simulink model "et_robocon_princess_pi"  (R2013b)
settings: Solver=FixedStepDiscrete  SolverMode=SingleTasking  StartTime=0.0  StopTime=inf  FixedStep=balancer_ts  RelTol=1e-3
undefined symbols (not defined in the file): a_d, a_r, balancerStates_Bus0, Batt, battery_gain, battery_offset, cmd_max, current_mode_status, current_task_operation_status, DiscIntNeverNeededParam, exec_period, Init_Bus0, K, k_f, k_i, k_phidot, k_thetadot, lightCalib, R, see_saw_princess, STATE, TRACK_MODE_LIST, ts2, W
libraries: legonxtlib x29, simulink x19, simulink_extras x4
(part 2 of 4)

== system et_robocon_princess_pi/Main Controller/normal_operation_modes.see_saw_princess/see_saw_mode.DispVar ==
  Var : Inport  OutDataTypeStr=single  PortDimensions=1
  f : TriggerPort  TriggerType=function-call
      settings: CopyFcn=Stateflow.SLINSF.SimulinkMan.removeBlockPreDeleteFcn  PreDeleteFcn=Stateflow.SLINSF.SimulinkMan.unsafePredeleteFcn
  Gain : Gain  Gain=100
  LCD : legonxtlib/LCD  slcdStr=Light  slcdLine=5  slcdFormat=Decimal
  wires:
  Var/1 -> Gain/1
  Gain/1 -> LCD/1

== system et_robocon_princess_pi/Main Controller/normal_operation_modes.see_saw_princess/see_saw_mode.Speak ==
  f : TriggerPort  TriggerType=function-call
      settings: CopyFcn=Stateflow.SLINSF.SimulinkMan.removeBlockPreDeleteFcn  PreDeleteFcn=Stateflow.SLINSF.SimulinkMan.unsafePredeleteFcn
  Constant : Constant  Value=50
  Speaker : legonxtlib/Speaker  sinputMode=Volume only  sspeakerFreq=800  sspeakerVolume=50  sspeakerDuration=100
  wires:
  Constant/1 -> Speaker/1

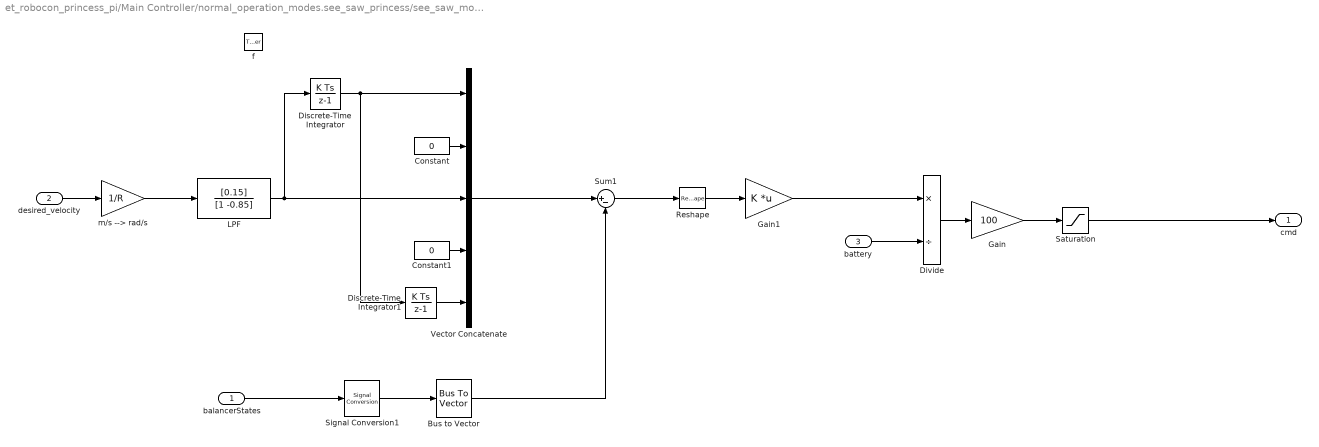
== system et_robocon_princess_pi/Main Controller/normal_operation_modes.see_saw_princess/see_saw_mode.balance_ctrl ==
  balancerStates : Inport  OutDataTypeStr=Bus: Balancer_States_Bus  PortDimensions=1
  desired_velocity : Inport  Port=2  OutDataTypeStr=single  PortDimensions=1  BusOutputAsStruct=on
  battery : Inport  Port=3  OutDataTypeStr=double  PortDimensions=1
  f : TriggerPort  TriggerType=function-call
      settings: CopyFcn=Stateflow.SLINSF.SimulinkMan.removeBlockPreDeleteFcn  PreDeleteFcn=Stateflow.SLINSF.SimulinkMan.unsafePredeleteFcn
  Bus to Vector : BusToVector
  Constant : Constant  Value=0  OutDataTypeStr=single
  Constant1 : Constant  Value=0  OutDataTypeStr=single
  Discrete-Time Integrator : DiscreteIntegrator  SampleTime=-1  ICPrevOutput=DiscIntNeverNeededParam  ICPrevScaledInput=DiscIntNeverNeededParam
  Discrete-Time Integrator1 : DiscreteIntegrator  SampleTime=-1  ICPrevOutput=DiscIntNeverNeededParam  ICPrevScaledInput=DiscIntNeverNeededParam
  Divide : Product  Inputs=*/
  Gain : Gain  Gain=100
  Gain1 : Gain  Gain=K  Multiplication=Matrix(K*u)
  LPF : DiscreteFilter  Numerator=[0.15]  Denominator=[1 -0.85]
  Reshape : Reshape  OutputDimensionality=Column vector (2-D)
  Saturation : Saturate  UpperLimit=100  LowerLimit=-100  OutDataTypeStr=single
  Signal Conversion1 : SignalConversion  ConversionOutput=Virtual bus
  Sum1 : Sum  Inputs=|+-
  Vector Concatenate : Concatenate  NumInputs=5
  m/s --> rad/s : Gain  Gain=1/R
  cmd : Outport  OutDataTypeStr=single  PortDimensions=1  InitialOutput=0
  wires:
  Reshape/1 -> Gain1/1
  Sum1/1 -> Reshape/1
  desired_velocity/1 -> m/s --> rad/s/1
  Bus to Vector/1 -> Sum1/2
  balancerStates/1 -> Signal Conversion1/1
  Vector Concatenate/1 -> Sum1/1
  battery/1 -> Divide/2
  Saturation/1 -> cmd/1
  Gain1/1 -> Divide/1
  Gain/1 -> Saturation/1
  Divide/1 -> Gain/1
  Signal Conversion1/1 -> Bus to Vector/1
  m/s --> rad/s/1 -> LPF/1
  Constant/1 -> Vector Concatenate/2
  LPF/1 -> Discrete-Time Integrator/1, Vector Concatenate/3
  Constant1/1 -> Vector Concatenate/4
  Discrete-Time Integrator/1 -> Discrete-Time Integrator1/1, Vector Concatenate/1
  Discrete-Time Integrator1/1 -> Vector Concatenate/5

== system et_robocon_princess_pi/Main Controller/normal_operation_modes.see_saw_princess/see_saw_mode.lineTracker ==
  desiredLight : Inport  OutDataTypeStr=single  PortDimensions=1
  light : Inport  Port=2  OutDataTypeStr=single  PortDimensions=1
  trackingPower : Inport  Port=3  OutDataTypeStr=single  PortDimensions=1
  battery : Inport  Port=4  OutDataTypeStr=double  PortDimensions=1
  f : TriggerPort  TriggerType=function-call
      settings: CopyFcn=Stateflow.SLINSF.SimulinkMan.removeBlockPreDeleteFcn  PreDeleteFcn=Stateflow.SLINSF.SimulinkMan.unsafePredeleteFcn
  Constant : Constant  Value=0  OutDataTypeStr=single
  Dead Zone : DeadZone  LowerValue=-0.02  UpperValue=0.02  SaturateOnIntegerOverflow=on
  Divide : Product  Inputs=*/
  Gain : Gain  Gain=100
  LPF and deriv : Subsystem
  PD : Gain  Gain="[4  0.02]/2"  Multiplication=Matrix(K*u)
  Product : Product
  Saturation : Saturate  UpperLimit=6  LowerLimit=-6
  Saturation1 : Saturate  UpperLimit=100  LowerLimit=-100  OutDataTypeStr=single
  Sum : Sum  Inputs=|+-
  Vector Concatenate : Concatenate
  Vector Concatenate1 : Concatenate
  switch side of line : Gain  Gain=-1
  cmd : Outport  OutDataTypeStr=single  PortDimensions=1
  wires:
  switch side of line/1 -> cmd/1
  desiredLight/1 -> Vector Concatenate/1
  Constant/1 -> Vector Concatenate/2  "desired light derivative"
  LPF and deriv/1(light_dot) -> Vector Concatenate1/2
  light/1 -> LPF and deriv/1(light), Vector Concatenate1/1
  Vector Concatenate/1 -> Sum/1
  Vector Concatenate1/1 -> Sum/2
  Sum/1 -> Dead Zone/1
  Dead Zone/1 -> PD/1
  PD/1 -> Saturation/1
  Saturation/1 -> Product/2
  trackingPower/1 -> Product/1
  Product/1 -> Divide/1
  battery/1 -> Divide/2
  Gain/1 -> Saturation1/1
  Divide/1 -> Gain/1
  Saturation1/1 -> switch side of line/1

== system et_robocon_princess_pi/Main Controller/normal_operation_modes.see_saw_princess/see_saw_mode.phiController ==
  phi : Inport  OutDataTypeStr=single  PortDimensions=1
  desiredPhi : Inport  Port=2  OutDataTypeStr=single  PortDimensions=1
  battery : Inport  Port=3  OutDataTypeStr=double  PortDimensions=1
  f : TriggerPort  TriggerType=function-call
      settings: CopyFcn=Stateflow.SLINSF.SimulinkMan.removeBlockPreDeleteFcn  PreDeleteFcn=Stateflow.SLINSF.SimulinkMan.unsafePredeleteFcn
  Divide : Product  Inputs=*/
  Gain : Gain  Gain=-10
  Gain1 : Gain  Gain=100
  Saturation1 : Saturate  UpperLimit=100  LowerLimit=-100  OutDataTypeStr=single
  Sum : Sum  Inputs=|+-
  cmd : Outport
  wires:
  desiredPhi/1 -> Sum/1
  phi/1 -> Sum/2
  Sum/1 -> Gain/1
  battery/1 -> Divide/2
  Gain1/1 -> Saturation1/1
  Divide/1 -> Gain1/1
  Gain/1 -> Divide/1
  Saturation1/1 -> cmd/1

== system et_robocon_princess_pi/Main Controller/normal_operation_modes.see_saw_princess/see_saw_mode.processLight ==
  rawLight : Inport  OutDataTypeStr=single  PortDimensions=1
  lightCalib : Inport  Port=2  OutDataTypeStr=Bus: Light_Bus  PortDimensions=1
  f : TriggerPort  TriggerType=function-call
      settings: CopyFcn=Stateflow.SLINSF.SimulinkMan.removeBlockPreDeleteFcn  PreDeleteFcn=Stateflow.SLINSF.SimulinkMan.unsafePredeleteFcn
  Bus Selector : BusSelector  OutputSignals=black,white
  Gain : Gain  Gain=0.3
  Gain1 : Gain  Gain=1/100
  Sum : Sum  Inputs=|+-
  Sum1 : Sum  Inputs=|++
  Sum2 : Sum  Inputs=|+-
  light : Outport
  wires:
  lightCalib/1 -> Bus Selector/1
  Bus Selector/1 -> Sum/1  "<black>"
  Bus Selector/2 -> Sum1/2, Sum/2  "<white>"
  Sum/1 -> Gain/1
  Gain/1 -> Sum1/1
  rawLight/1 -> Sum2/1
  Sum1/1 -> Sum2/2
  Sum2/1 -> Gain1/1
  Gain1/1 -> light/1

== system et_robocon_princess_pi/Main Controller/normal_operation_modes.see_saw_princess/see_saw_mode.tail_controller ==
  note: Could be improved, PI for example
  current : Inport  OutDataTypeStr=single  PortDimensions=1
  desired : Inport  Port=2  OutDataTypeStr=single  PortDimensions=1
  f : TriggerPort  TriggerType=function-call
      settings: CopyFcn=Stateflow.SLINSF.SimulinkMan.removeBlockPreDeleteFcn  PreDeleteFcn=Stateflow.SLINSF.SimulinkMan.unsafePredeleteFcn
  Gain : Gain  Gain=250
  Saturation : Saturate  UpperLimit=100  LowerLimit=-100  OutDataTypeStr=single
  Sum : Sum  Inputs=|+-
  cmd : Outport  OutDataTypeStr=single  PortDimensions=1  InitialOutput=0
  wires:
  Sum/1 -> Gain/1
  current/1 -> Sum/2
  desired/1 -> Sum/1
  Gain/1 -> Saturation/1
  Saturation/1 -> cmd/1

== system et_robocon_princess_pi/State Estimation/Data Type Conversion Unit Conversion Tail Initialization ==
  u : Inport
  init_tail : Inport  Port=2
  Bus Creator : BusCreator  Inputs=11  OutDataTypeStr=Bus: Sensors_Bus
  Bus Selector : BusSelector  OutputSignals=theta_L,theta_R,theta_T,light,gyro,sonar,battery,touch,time,ok_button,BT_status_in
  Degrees to Radians{,1..2,4} (4 alike) : simulink_extras/Transformations/Degrees to Radians
  Low Pass Filter : Subsystem
  Process Sonar : Subsystem  Commented=through
  Vmax : Subsystem
  tail processing : Subsystem
  y : Outport
  wires:
  Bus Selector/11 -> Bus Creator/11  "<BT_status_in>"
  Process Sonar/1(sonar) -> Bus Creator/6
  Bus Selector/6 -> Process Sonar/1(sonar_in)  "<sonar>"
  Bus Selector/10 -> Bus Creator/10  "<ok_button>"
  init_tail/1 -> tail processing/2(init_tail)
  Bus Selector/9 -> Bus Creator/9  "<time>"
  Bus Selector/8 -> Bus Creator/8  "<touch>"
  tail processing/1(tail) -> Bus Creator/3  "theta_T"
  Degrees to Radians4/1 -> tail processing/1(sensors)
  Vmax/1(Vmax) -> Bus Creator/7  "battery"
  Degrees to Radians2/1 -> Bus Creator/5  "gyro"
  Bus Selector/3 -> Degrees to Radians4/1  "<theta_T>"
  Bus Selector/7 -> Low Pass Filter/1(u)  "<battery>"
  Bus Selector/5 -> Degrees to Radians2/1  "<gyro>"
  Bus Selector/4 -> Bus Creator/4  "<light>"
  Bus Creator/1 -> y/1
  u/1 -> Bus Selector/1
  Degrees to Radians/1 -> Bus Creator/1  "theta_L"
  Bus Selector/2 -> Degrees to Radians1/1  "<theta_R>"
  Bus Selector/1 -> Degrees to Radians/1  "<theta_L>"
  Low Pass Filter/1(y) -> Vmax/1(Battery)  "battery"
  Degrees to Radians1/1 -> Bus Creator/2  "theta_R"

== system et_robocon_princess_pi/State Estimation/Fall Detection ==
  gyro : Inport
      settings: AttributesFormatString=Output data type: %<OutDataTypeStr>
  reset : Inport  Port=2  OutDataTypeStr=boolean
      settings: AttributesFormatString=Output data type: %<OutDataTypeStr>
  Abs : Abs
  Compare To Constant : simulink/Logic and Bit Operations/Compare To Constant  relop=>  const=1  OutDataTypeStr=boolean
  Terminator : Terminator
  aggregate_fall_detection_comparison : Logic  Operator=OR  OutDataTypeStr=boolean
  boolean_to_integer_conversion : DataTypeConversion  OutDataTypeStr=uint8
      settings: AttributesFormatString=Output data type: %<OutDataTypeStr>
  previous_fall_detection_status : UnitDelay  SampleTime=-1
  reset_output_overrice_switch : MultiPortSwitch  DataPortOrder=Zero-based contiguous  Inputs=2  zeroidx=on  InputSameDT=on
  reset_output_value : Constant  Value=false
  reset_output_value1 : Constant  Value=false  OutDataTypeStr=boolean
  fall_detected : Outport
  wires:
  reset_output_overrice_switch/1 -> Terminator/1, previous_fall_detection_status/1
  reset_output_value/1 -> reset_output_overrice_switch/3
  aggregate_fall_detection_comparison/1 -> reset_output_overrice_switch/2
  boolean_to_integer_conversion/1 -> reset_output_overrice_switch/1
  reset/1 -> boolean_to_integer_conversion/1
  previous_fall_detection_status/1 -> aggregate_fall_detection_comparison/2
  Abs/1 -> Compare To Constant/1
  gyro/1 -> Abs/1
  Compare To Constant/1 -> aggregate_fall_detection_comparison/1
  reset_output_value1/1 -> fall_detected/1

== stateflow chart et_robocon_princess_pi/Main Controller ==
  state restore
  state emergency_stop
    entry:
    debugFlag = uint16(9999);
  state normal_operation_modes
    state gyro_calibration_mode
    state light_calibration_up
    state line_tracking_mode
    state see_saw_princess
    state line_tracking_after_seesaw
    state WeShouldNotBeHere
    (default) -> (junction 12) : {
        | current_mode_status = OperationModeStatusEnum.IN_PROGRESS;
        | }
    (junction 12) -> gyro_calibration_mode [order 1] : [  current_mode == OperationModeEnum.GYRO_CALIBRATION ]
    (junction 12) -> (junction 13) [order 2]
    (junction 13) -> ? [order 1] : [ current_mode == OperationModeEnum.LIGHT_CALIBRATION_ON_TAIL ]
    (junction 13) -> (junction 144) [order 1]
    (junction 144) -> light_calibration_up [order 1] : [ current_mode == OperationModeEnum.LIGHT_CALIBRATION_UP ]
    (junction 144) -> (junction 14) [order 2]
    (junction 14) -> line_tracking_mode [order 1] : [ current_mode == OperationModeEnum.LINE_TRACKING ]
    (junction 14) -> (junction 15) [order 2]
    (junction 15) -> see_saw_princess [order 1] : [ current_mode == OperationModeEnum.SEE_SAW_PRINCESS ]
    (junction 15) -> (junction 17) [order 2]
    (junction 17) -> ? [order 1] : [  current_mode == OperationModeEnum.LIMBO ]
    (junction 17) -> (junction 19) [order 1]
    (junction 19) -> ? [order 1] : [ current_mode == OperationModeEnum.LIGHT_CALIBRATION_LIMBO ]
    (junction 19) -> (junction 140) [order 1]
    (junction 140) -> line_tracking_after_seesaw [order 1] : [ current_mode == OperationModeEnum.LINE_TRACKING_ON_MAP ]
    (junction 140) -> (junction 154) [order 2]
    (junction 154) -> ? [order 1] : [ current_mode == OperationModeEnum.YOSHI ]
    (junction 154) -> (junction 99) [order 1]
    (junction 99) -> WeShouldNotBeHere
  (default) -> (junction 38) : {initFlags = Init_Bus0;BT_status_out = single(0)}
  (junction 37) -> (junction 38)
  (junction 43) -> (junction 37)
  (junction 38) -> (junction 39) : { current_mode_index = uint8( 0 ); }
  (junction 40) -> (junction 39)
  restore -> (junction 40) : [ false == touch ]
  (junction 39) -> (junction 41) : {
      | current_mode_status = OperationModeStatusEnum.NOT_STARTED;
      | }
  normal_operation_modes -> (junction 40) [order 2] : [ current_mode_status == OperationModeStatusEnum.SUCCESSFULLY_COMPLETED ]
  (junction 42) -> (junction 41)
  (junction 41) -> (junction 44) : { current_mode_index = current_mode_index + uint8( 1 ); }
  (junction 47) -> (junction 42)
  emergency_stop -> restore : [ true == touch ]
  (junction 44) -> (junction 43) [order 1] : [ numel( TRACK_MODE_LIST ) < current_mode_index ]
      | % If the "current_mode_index" has exceeded the number
      | % of elements in the list, it should "wrap" back to the start.
  (junction 44) -> (junction 45) [order 2]
  (junction 45) -> (junction 46) : {
      | current_mode = TRACK_MODE_LIST( current_mode_index );
      | }
  (junction 46) -> (junction 47) [order 1] : [  current_mode == OperationModeEnum.SKIP ]
  (junction 46) -> normal_operation_modes [order 2]
  normal_operation_modes -> emergency_stop [order 1] : [ true == fall_detection_input ]
      | {current_mode_status = OperationModeStatusEnum.ABORTED;}
  data: rawSensors input Bus: Sensors_Bus size=1; PWM output Bus: PWM_bus size=1; TRACK_MODE_LIST parameter Enum: OperationModeEnum; current_mode_index local uint8; current_mode data_store_memory; states input Bus: States_Bus size=1; fall_detection_input input boolean size=1; current_mode_status data_store_memory; sensors input Bus: Sensors_Bus size=1; lightCalib data_store_memory; debugFlag output uint16 size=1; BT_status_out output single size=1; touch input single size=1; initFlags output Bus: Init_Bus size=1; Init_Bus0 parameter Bus: Init_Bus size=1; balancerStates_Bus0 parameter Bus: Balancer_States_Bus size=1

== stateflow chart et_robocon_princess_pi/Main Controller/normal_operation_modes.light_calibration_up ==
  state wait
    entry:debugFlag = uint16(200);
  state MoveUp
    entry:debugFlag = uint16(201);
    PWM.tail = single(-50);
  state Reset
    entry:debugFlag = uint16(202);
    PWM.tail = single(0);
    initFlags.tail = single(1);
    exit:
    initFlags.tail = single(0);
    desired_tail = single(0);
  state light_sensor_calibration_up
    %during, exit: PWM.tail = tail_controller(sensors.theta_T,single(1.6))
    state WaitForBlack
      entry: debugFlag = uint16(310);
    state StoreBlack
      entry: lightCalib.black = sensors.light;
      debugFlag = uint16(311);
    state WaitForWhite
      entry: debugFlag = uint16(312)
    state StoreWhite
      entry: lightCalib.white = sensors.light;
      debugFlag = uint16(313);
    state CalibComplete
      entry:
      debugFlag = uint16(318);
      current_task_operation_status = OperationModeStatusEnum.SUCCESSFULLY_COMPLETED;
    state cmd = tail_controller(current,desired) [function]
    (default) -> WaitForBlack
    WaitForBlack -> StoreBlack : [hasChangedFrom(touch,single(0))]
    StoreBlack -> WaitForWhite : after(1,sec)
    WaitForWhite -> StoreWhite : [hasChangedFrom(touch,single(0))]
    StoreWhite -> CalibComplete : after(1,sec)
  (default) -> wait
  wait -> MoveUp : [hasChangedFrom(touch,single(0))]
  MoveUp -> Reset : after(2,sec)
  Reset -> light_sensor_calibration_up : after(1,sec)
  data: current function_input single size=1; desired function_input single size=1; cmd function_output single size=1; sensors input Bus: Sensors_Bus size=1; lightCalib data_store_memory; current_task_operation_status data_store_memory; debugFlag output uint16; touch input single size=1; PWM output Bus: PWM_bus size=1; initFlags output Bus: Init_Bus size=1; desired_tail local

== stateflow chart et_robocon_princess_pi/Main Controller/normal_operation_modes.gyro_calibration_mode ==
  state gyro_calibration_mode
    state GyroCalibration
      entry:
      desired_tail = single(1.6);
      during, exit:
      PWM.tail = tail_controller(sensors.theta_T,desired_tail);
      state MoveTailDown
        entry:
        debugFlag = uint16(204);
        during:
        desired_tail = desired_tail + single(0.008);
      state StartCalibration
        entry:
        debugFlag = uint16(205);
        initFlags.gyroInit = single(1);
        initFlags.gyroReset = single(1);
        initFlags.theta = single(1);
      state Wait
        entry: Speak;
      state MakeNoise
        during: Speak;
      state StartCalibration1
        entry:
        debugFlag = uint16(208);
        initFlags.gyroInit = single(0);
        initFlags.gyroReset = single(0);
        initFlags.theta = single(0);
      state CalibComplete
        entry:
        debugFlag = uint16(209);
        current_task_operation_status = OperationModeStatusEnum.SUCCESSFULLY_COMPLETED;
      state cmd = tail_controller(current,desired) [function]
      state Speak [function]
      (default) -> StartCalibration
      MoveTailDown -> StartCalibration : [desired_tail >= single(1.6) ]
      StartCalibration -> Wait : [hasChangedFrom(touch,single(0))]
      Wait -> MakeNoise : after(5,sec)
      MakeNoise -> StartCalibration1 : after(0.5,sec)
      StartCalibration1 -> CalibComplete
    (default) -> GyroCalibration
  data: current function_input single size=1; desired function_input single size=1; cmd function_output single size=1; debugFlag output uint16 size=1; current_task_operation_status data_store_memory; sensors input Bus: Sensors_Bus size=1; touch input single size=1; initFlags output Bus: Init_Bus size=1; PWM output Bus: PWM_bus size=1; desired_tail local

== system et_robocon_princess_pi/State Estimation/Gyro Processing ==
  sensors : Inport
  gyroInit : Inport  Port=2
  gyroReset : Inport  Port=3
  Bus Selector1 : BusSelector  OutputSignals=gyro
  Compute psi : Subsystem
  Gyro initialization : Subsystem  TreatAsAtomicUnit=on
  Reset Subsystem : Stateflow chart  TreatAsAtomicUnit=on
  Sum : Sum  Inputs=-+|
  psi : Outport
  psi_dot : Outport  Port=2
  psi filtered : Outport  Port=3
  wires:
  Compute psi/2(Filtered) -> psi filtered/1
  Reset Subsystem/1(doProcess()) -> Compute psi/Trigger
  gyroReset/1 -> Reset Subsystem/1(init_flag)
  Bus Selector1/1 -> Sum/2, Gyro initialization/1(gyro)  "<gyro>"
  Gyro initialization/1(psi_dot_0) -> Sum/1
  Sum/1 -> psi_dot/1, Compute psi/1(gyro)
  Compute psi/1(psi) -> psi/1
  sensors/1 -> Bus Selector1/1
  gyroInit/1 -> Gyro initialization/Enable

== system et_robocon_princess_pi/State Estimation/StateEstimation ==
  note: Conversion from Raw Sensors to States as described in "NXTway plant model.pdf"
  Sensors : Inport
  psi : Inport  Port=2
  psi_dot : Inport  Port=3
  init theta : Inport  Port=4
  Bus Creator1 : BusCreator  OutDataTypeStr=Bus: States_Bus
  Bus Creator2 : BusCreator  Inputs=5  OutDataTypeStr=Bus: Balancer_States_Bus
  Bus Selector1 : BusSelector  OutputSignals=theta_L,theta_R
  Process theta1 : Subsystem
  Reset Subsystem : Stateflow chart  TreatAsAtomicUnit=on
  states : Outport  OutputWhenDisabled=reset  InitialOutput=0
  wires:
  Process theta1/2(psi_out) -> Bus Creator2/2  "psi"
  Reset Subsystem/1(doProcess()) -> Process theta1/Trigger
  Bus Selector1/2 -> Process theta1/3(theta_r)  "<theta_R>"
  Bus Selector1/1 -> Process theta1/2(theta_l)  "<theta_L>"
  init theta/1 -> Reset Subsystem/1(init_flag)
  Process theta1/1(theta) -> Bus Creator2/1
  Process theta1/3(theta_dot) -> Bus Creator2/3
  Process theta1/4(int_theta) -> Bus Creator2/5
  psi_dot/1 -> Bus Creator2/4  "psi_dot"
  Process theta1/6(phi_dot) -> Bus Creator1/3  "phi_dot"
  Bus Creator2/1 -> Bus Creator1/1  "balancerStates"
  Process theta1/5(phi) -> Bus Creator1/2  "phi"
  Sensors/1 -> Bus Selector1/1
  psi/1 -> Process theta1/1(psi)
  Bus Creator1/1 -> states/1
  Process theta1/7(theta_dot_dot) -> Bus Creator1/4  "theta_dot_dot"

== system et_robocon_princess_pi/Hardware/Receive Bluetooth Status/BluetoothOFF ==
  Constant : Constant  Value=single(0)
  BT_status_in : Outport
  wires:
  Constant/1 -> BT_status_in/1

== system et_robocon_princess_pi/Hardware/Receive Bluetooth Status/BluetoothONMario ==
  Data Type Conversion9 : DataTypeConversion  OutDataTypeStr=single
  Rate Transition2 : RateTransition  OutPortSampleTime=0.004
  Receive via Bluetooth(R) Connection : legonxtlib/Receive via Bluetooth(R) Connection  mailbox=3  dataType=uint8  dataSize=1  sampleTime=0.1
  Terminator : Terminator
  BT_status_in : Outport
  wires:
  Data Type Conversion9/1 -> BT_status_in/1
  Rate Transition2/1 -> Data Type Conversion9/1
  Receive via Bluetooth(R) Connection/1 -> Rate Transition2/1
  Receive via Bluetooth(R) Connection/2 -> Terminator/1

== system et_robocon_princess_pi/Hardware/Receive Bluetooth Status/BluetoothONPrincess ==
  Data Type Conversion9 : DataTypeConversion  OutDataTypeStr=single
  Rate Transition2 : RateTransition  OutPortSampleTime=0.004
  Receive via Bluetooth(R) Connection : legonxtlib/Receive via Bluetooth(R) Connection  mailbox=3  dataType=uint8  dataSize=1  sampleTime=0.1
  Terminator : Terminator
  BT_status_in : Outport
  wires:
  Receive via Bluetooth(R) Connection/2 -> Terminator/1
  Receive via Bluetooth(R) Connection/1 -> Rate Transition2/1
  Rate Transition2/1 -> Data Type Conversion9/1
  Data Type Conversion9/1 -> BT_status_in/1

== system et_robocon_princess_pi/Hardware/Send Bluetooth Status/BluetoothOFF ==
  BT_status_out : Inport
  Terminator : Terminator
  wires:
  BT_status_out/1 -> Terminator/1

== system et_robocon_princess_pi/Hardware/Send Bluetooth Status/BluetoothONMario ==
  BT_status_out : Inport
  Data Type Conversion1 : DataTypeConversion  OutDataTypeStr=uint8
  Rate Transition1 : RateTransition  OutPortSampleTime=0.1
  Send via Bluetooth(R) Connection : legonxtlib/Send via Bluetooth(R) Connection  mailbox=2
  wires:
  BT_status_out/1 -> Rate Transition1/1
  Rate Transition1/1 -> Data Type Conversion1/1
  Data Type Conversion1/1 -> Send via Bluetooth(R) Connection/1

== system et_robocon_princess_pi/Hardware/Send Bluetooth Status/BluetoothONPrincess ==
  BT_status_out : Inport
  Data Type Conversion1 : DataTypeConversion  OutDataTypeStr=uint8
  Rate Transition1 : RateTransition  OutPortSampleTime=0.1
  Send via Bluetooth(R) Connection : legonxtlib/Send via Bluetooth(R) Connection  mailbox=4
  wires:
  Data Type Conversion1/1 -> Send via Bluetooth(R) Connection/1
  Rate Transition1/1 -> Data Type Conversion1/1
  BT_status_out/1 -> Rate Transition1/1

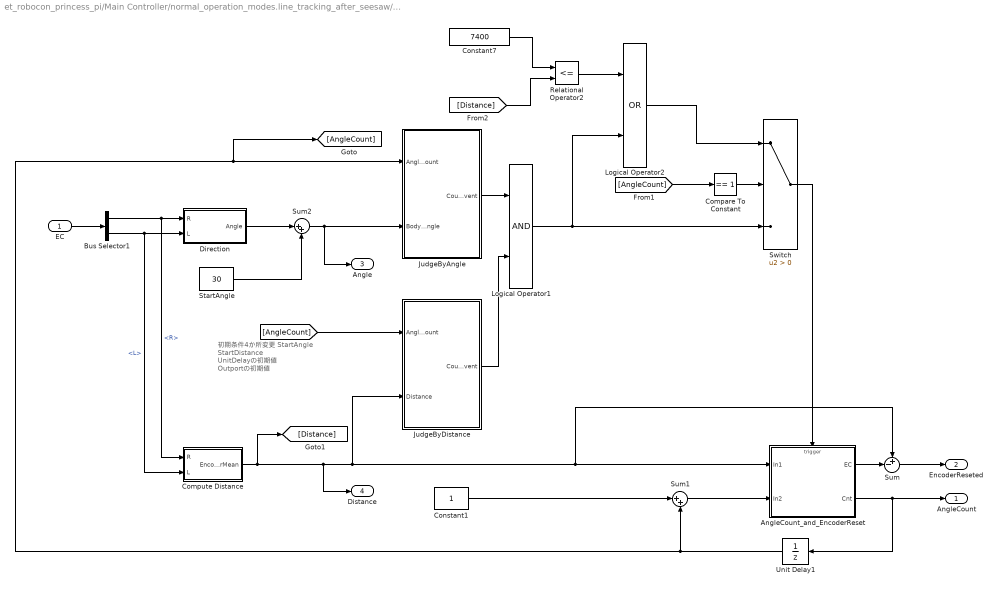
== system et_robocon_princess_pi/Main Controller/normal_operation_modes.line_tracking_after_seesaw/line_tracking_mode.Track.analyzeEncoders/AngleCounter ==
  note: 初期条件4か所変更
      | StartAngle
      | StartDistance
      | UnitDelayの初期値
      | Outportの初期値
  EC : Inport
  AngleCount_and_EncoderReset : Subsystem  TreatAsAtomicUnit=on
  Bus Selector1 : BusSelector  OutputSignals=R,L
  Compare To Constant : simulink/Logic and Bit Operations/Compare To Constant  relop===  const=1  OutDataTypeStr=boolean
  Compute Distance : Subsystem
  Constant1 : Constant  OutDataTypeStr=uint8
  Constant7 : Constant  Value=7400  OutDataTypeStr=int32
  Direction : Subsystem
  JudgeByAngle : Subsystem
  JudgeByDistance : Subsystem
  Logical Operator1 : Logic  AllPortsSameDT=off  OutDataTypeStr=boolean
  Logical Operator2 : Logic  Operator=OR  AllPortsSameDT=off  OutDataTypeStr=boolean
  Relational Operator2 : RelationalOperator  Operator=<=  OutDataTypeStr=boolean
  StartAngle : Constant  Value=30  OutDataTypeStr=int16
  Sum : Sum  Inputs=+-|
  Sum1 : Sum  Inputs=|++  AccumDataTypeStr=uint8
  Sum2 : Sum  Inputs=|++
  Switch : Switch  Criteria=u2 > Threshold
  Unit Delay1 : UnitDelay  InitialCondition=1  SampleTime=-1
  AngleCount : Outport
  EncoderReseted : Outport  Port=2
  Angle : Outport  Port=3
  Distance : Outport  Port=4
  wires:
  Sum2/1 -> JudgeByAngle/2(BodyAngle), Angle/1
  Sum1/1 -> AngleCount_and_EncoderReset/2(In2)
  Constant1/1 -> Sum1/1
  Unit Delay1/1 -> [AngleCount], JudgeByAngle/1(AngleCount), Sum1/2
  AngleCount_and_EncoderReset/2(Cnt) -> AngleCount/1, Unit Delay1/1
  Bus Selector1/1 -> Compute Distance/1(R), Direction/1(R)  "<R>"
  Bus Selector1/2 -> Compute Distance/2(L), Direction/2(L)  "<L>"
  EC/1 -> Bus Selector1/1
  AngleCount_and_EncoderReset/1(EC) -> Sum/2
  Sum/1 -> EncoderReseted/1
  Compute Distance/1(EncoderMean) -> [Distance], Distance/1, JudgeByDistance/2(Distance), Sum/1, AngleCount_and_EncoderReset/1(In1)
  [AngleCount] -> JudgeByDistance/1(AngleCount)
  JudgeByAngle/1(CountEvent) -> Logical Operator1/1
  JudgeByDistance/1(CountEvent) -> Logical Operator1/2
  Direction/1(Angle) -> Sum2/1
  StartAngle/1 -> Sum2/2
  Logical Operator1/1 -> Logical Operator2/2, Switch/3
  Switch/1 -> AngleCount_and_EncoderReset/Trigger
  Compare To Constant/1 -> Switch/2
  [AngleCount] -> Compare To Constant/1
  Logical Operator2/1 -> Switch/1
  Constant7/1 -> Relational Operator2/1
  Relational Operator2/1 -> Logical Operator2/1
  [Distance] -> Relational Operator2/2

== system et_robocon_princess_pi/Main Controller/normal_operation_modes.line_tracking_after_seesaw/line_tracking_mode.Track.analyzeEncoders/Store x0 ==
  In1 : Inport
  In2 : Inport  Port=2
  Enable : EnablePort
  Out1 : Outport
  Out2 : Outport  Port=2
  wires:
  In1/1 -> Out1/1
  In2/1 -> Out2/1

== system et_robocon_princess_pi/Main Controller/normal_operation_modes.line_tracking_after_seesaw/line_tracking_mode.Track.lineTracker/Handler ==
  steering : Inport
  fwd : Inport  Port=2
  Constant1 : Constant  Value=-1  OutDataTypeStr=int8
  Mux : Mux  Inputs=2
  Switch1 : Switch  OutDataTypeStr=single  RndMeth=Simplest
  rocket_start : Subsystem
  slow_start : Subsystem
  cmd : Outport
  wires:
  steering/1 -> Mux/2  "str"
  slow_start/1(fwd_slow) -> Switch1/1
  Mux/1 -> cmd/1
  fwd/1 -> rocket_start/1(fwd), slow_start/1(fwd)  "fwd"
  Constant1/1 -> Switch1/2
  rocket_start/1(fwd_slow) -> Switch1/3
  Switch1/1 -> Mux/1

== system et_robocon_princess_pi/Main Controller/normal_operation_modes.line_tracking_after_seesaw/line_tracking_mode.Track.lineTracker/SwitchForFreeSteering ==
  note: Edge Change
      | -1: Run right edge
      | 1: Run left edge
  note: Target Value
  FlagSteering : Inport
  PID : Inport  Port=2  PortDimensions=5
  LightSens : Inport  Port=3
  Add : Sum  Inputs=+-  AccumDataTypeStr=single  OutDataTypeStr=single  RndMeth=Simplest
  AdjustForUnit : Gain  Gain=18.25  OutDataTypeStr=single  RndMeth=Simplest
  Constant2 : Constant  OutDataTypeStr=single  SampleTime=-1
  Constant6 : Constant  Value=0.5  OutDataTypeStr=single  SampleTime=-1
  DeleteDummyData : Selector  InputPortWidth=5  IndexOptions=Index vector (dialog)  Indices=1  OutputSizes=1
  Product1 : Product  OutDataTypeStr=single  RndMeth=Simplest
  Switch : Switch  Criteria=u2 > Threshold
  tmpController : Subsystem  TreatAsAtomicUnit=on  mask(tmp PID Controller){Ts_=ts2, SaturationMax=100, SaturationMin=-100}
      mask prompts: Ts_ "Sampling Time (Task Period)"; SaturationMax "Saturation Max Value of PID Ctrl"; SaturationMin "Saturation Min Value of PID"
      mask help:
      | Sampling Time: Task Period
      | P: Proportional Gain
      | I: Integral Gain
      | D: Derivative Gain
      | B: Back Gain for Integrator
      | Saturation Max Value of PID ctrl:
      |    Saturation Max Value of PID ctrl > Saturation Min Value of PID ctrl
      | Saturation Min Value of PID ctrl:
      |    Saturation Min Value of PID ctrl < Saturation Max Value of PID ctrl
      settings: RTWSystemCode=Inline
      mask Display: disp('PID')
  Steering : Outport
  wires:
  PID/1 -> tmpController/2(BD), DeleteDummyData/1
  Switch/1 -> Steering/1
  DeleteDummyData/1 -> Switch/1  "FreeSteering"
  FlagSteering/1 -> Switch/2
  Add/1 -> Product1/1
  LightSens/1 -> Add/1
  Constant6/1 -> Add/2
  Constant2/1 -> Product1/2
  Product1/1 -> tmpController/1(Error)  "Diff_Between_Target_and_Value"
  tmpController/1(Target_deg) -> AdjustForUnit/1
  AdjustForUnit/1 -> Switch/3  "LintTraceSteering"

== system et_robocon_princess_pi/Main Controller/normal_operation_modes.line_tracking_after_seesaw/line_tracking_mode.Track.processLight/OFF2ON ==
  In1 : Inport
  Trigger : TriggerPort
  Light Sensor Switch ON : S-Function  FunctionName=sfun_light_sw  Parameters=-1,ip,sw  EnableBusSupport=off  mask(Light Sensor ON/OFF Switch){ip=S3, sw=ON}
      mask prompts: ip "port:"; sw "switch"
      mask help: LEGO Mindstorms NXT Light Sensor switch.
      mask init:
      | [data, map]=imread('LIGHT_SENSOR.gif');
      | pic=ind2rgb(data,map);
      mask TypeOptions ip: S1 | S2 | S3 | S4
      mask TypeOptions sw: ON | OFF
      mask Display:
      | image(pic)
      | color('red')
      | fprintf('%s, %s',ip,sw)
  Out1 : Outport
  wires:
  In1/1 -> Out1/1

== system et_robocon_princess_pi/Main Controller/normal_operation_modes.line_tracking_after_seesaw/line_tracking_mode.Track.processLight/ON2OFF ==
  In1 : Inport
  Trigger : TriggerPort  TriggerType=falling
  Light Sensor Switch OFF : S-Function  FunctionName=sfun_light_sw  Parameters=-1,ip,sw  EnableBusSupport=off  mask(Light Sensor ON/OFF Switch){ip=S3, sw=OFF}
      mask prompts: ip "port:"; sw "switch"
      mask help: LEGO Mindstorms NXT Light Sensor switch.
      mask init:
      | [data, map]=imread('LIGHT_SENSOR.gif');
      | pic=ind2rgb(data,map);
      mask TypeOptions ip: S1 | S2 | S3 | S4
      mask TypeOptions sw: ON | OFF
      mask Display:
      | image(pic)
      | color('red')
      | fprintf('%s, %s',ip,sw)
  Out1 : Outport
  wires:
  In1/1 -> Out1/1

== system et_robocon_princess_pi/Main Controller/normal_operation_modes.line_tracking_after_seesaw/line_tracking_mode.balanceControl/ForSimulation ==
  cmd_forward : Inport
  cmd_turn : Inport  Port=2
  gyro : Inport  Port=3
  gyro_offset : Inport  Port=4
  theta_m_l : Inport  Port=5
  theta_m_r : Inport  Port=6
  battery : Inport  Port=7
  Cal_PWM : Subsystem
      settings: RTWSystemCode=Nonreusable function
  Cal_Reference : Subsystem  Description=|
      | 1111111111111111111
      | 2222222222222222222
      | 3333333333333333333
      | 4444444444444444444
      settings: RTWSystemCode=Nonreusable function
  Cal_x1 : Subsystem
      settings: RTWSystemCode=Nonreusable function
  DiscreteIntegrator : Subsystem
  FeedbackGain : Gain  Gain=k_f  Multiplication=Matrix(K*u)  OutDataTypeStr=Inherit: Same as input  ParamDataTypeStr=Inherit: Same as input
  IntegralGain : Gain  Gain=k_i  Multiplication=Matrix(K*u)  OutDataTypeStr=Inherit: Same as input  ParamDataTypeStr=Inherit: Same as input
  Sum1 : Sum  Inputs=|+-  OutDataTypeStr=Inherit: Same as first input
  Sum2 : Sum  Inputs=+-|  OutDataTypeStr=Inherit: Same as first input
  sum_err : Sum  Inputs=|++  OutDataTypeStr=Inherit: Same as first input
  pwm_l : Outport
  pwm_r : Outport  Port=2
  wires:
  Cal_Reference/1(pwm_turn) -> Cal_PWM/1(pwm_turn)
  cmd_turn/1 -> Cal_Reference/2(cmd_turn)
  sum_err/1 -> Cal_PWM/2(err)
  FeedbackGain/1 -> sum_err/2  "errx1"
  Cal_Reference/2(theta_ref) -> Sum1/1
  Cal_x1/1(theta) -> Sum1/2
  Sum1/1 -> DiscreteIntegrator/1(in)
  DiscreteIntegrator/1(out) -> IntegralGain/1
  IntegralGain/1 -> sum_err/1  "errtheta"
  Cal_x1/2(x1) -> Sum2/2
  Sum2/1 -> FeedbackGain/1
  Cal_Reference/3(x1_ref) -> Sum2/1
  theta_m_l/1 -> Cal_x1/3(theta_m_l)
  theta_m_r/1 -> Cal_x1/4(theta_m_r)
  cmd_forward/1 -> Cal_Reference/1(cmd_forward)
  Cal_PWM/1(pwm_l) -> pwm_l/1
  gyro/1 -> Cal_x1/1(gyro)
  Cal_PWM/2(pwm_r) -> pwm_r/1
  gyro_offset/1 -> Cal_x1/2(gyro_offset)
  battery/1 -> Cal_PWM/3(battery)

== system et_robocon_princess_pi/Main Controller/normal_operation_modes.line_tracking_after_seesaw/line_tracking_mode.balanceControl/Low Pass Filter ==
  u : Inport
  Constant : Constant  Value=0  OutDataTypeStr=boolean
  Low Pass Filter : DiscreteFilter  Numerator=[.01]  Denominator=[1 -0.99]
  Memory : Memory  X0=1  InheritSampleTime=on
  Store Offset : Subsystem  TreatAsAtomicUnit=on
  Sum1 : Sum  Inputs=++|
  Sum2 : Sum  Inputs=-+|
  y : Outport
  wires:
  Store Offset/1(x0) -> Sum1/1, Sum2/1
  u/1 -> Store Offset/1(x), Sum2/2
  Constant/1 -> Memory/1
  Memory/1 -> Store Offset/Enable
  Sum2/1 -> Low Pass Filter/1
  Sum1/1 -> y/1
  Low Pass Filter/1 -> Sum1/2

== system et_robocon_princess_pi/Main Controller/normal_operation_modes.line_tracking_after_seesaw/line_tracking_mode.balanceControl/removeOffset ==
  In1 : Inport
  In2 : Inport  Port=2
  Constant : Constant  Value=0
  Memory : Memory  X0=1  InheritSampleTime=on
  Store x0 : Subsystem  TreatAsAtomicUnit=on
  Sum : Sum  Inputs=-+|
  Sum1 : Sum  Inputs=-+|
  Out1 : Outport
  Out2 : Outport  Port=2
  wires:
  Store x0/2(Out2) -> Sum1/1
  In2/1 -> Store x0/2(In2), Sum1/2
  Constant/1 -> Memory/1
  Sum1/1 -> Out2/1
  In1/1 -> Sum/2, Store x0/1(In1)
  Store x0/1(Out1) -> Sum/1
  Memory/1 -> Store x0/Enable
  Sum/1 -> Out1/1

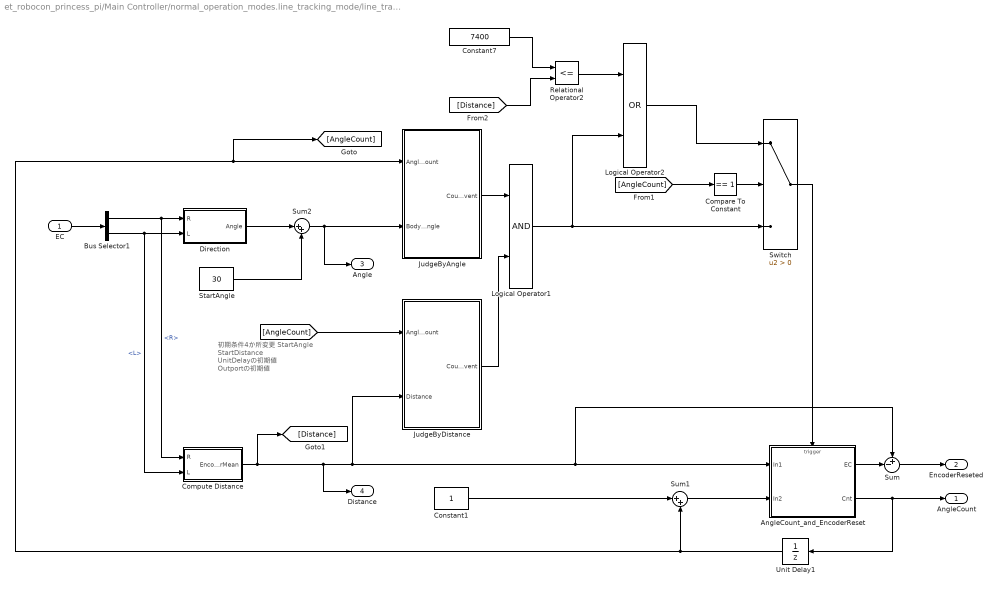
== system et_robocon_princess_pi/Main Controller/normal_operation_modes.line_tracking_mode/line_tracking_mode.Track.analyzeEncoders/AngleCounter ==
  note: 初期条件4か所変更
      | StartAngle
      | StartDistance
      | UnitDelayの初期値
      | Outportの初期値
  EC : Inport
  AngleCount_and_EncoderReset : Subsystem  TreatAsAtomicUnit=on
  Bus Selector1 : BusSelector  OutputSignals=R,L
  Compare To Constant : simulink/Logic and Bit Operations/Compare To Constant  relop===  const=1  OutDataTypeStr=boolean
  Compute Distance : Subsystem
  Constant1 : Constant  OutDataTypeStr=uint8
  Constant7 : Constant  Value=7400  OutDataTypeStr=int32
  Direction : Subsystem
  JudgeByAngle : Subsystem
  JudgeByDistance : Subsystem
  Logical Operator1 : Logic  AllPortsSameDT=off  OutDataTypeStr=boolean
  Logical Operator2 : Logic  Operator=OR  AllPortsSameDT=off  OutDataTypeStr=boolean
  Relational Operator2 : RelationalOperator  Operator=<=  OutDataTypeStr=boolean
  StartAngle : Constant  Value=30  OutDataTypeStr=int16
  Sum : Sum  Inputs=+-|
  Sum1 : Sum  Inputs=|++  AccumDataTypeStr=uint8
  Sum2 : Sum  Inputs=|++
  Switch : Switch  Criteria=u2 > Threshold
  Unit Delay1 : UnitDelay  InitialCondition=1  SampleTime=-1
  AngleCount : Outport
  EncoderReseted : Outport  Port=2
  Angle : Outport  Port=3
  Distance : Outport  Port=4
  wires:
  Sum2/1 -> JudgeByAngle/2(BodyAngle), Angle/1
  Sum1/1 -> AngleCount_and_EncoderReset/2(In2)
  Constant1/1 -> Sum1/1
  Unit Delay1/1 -> [AngleCount], JudgeByAngle/1(AngleCount), Sum1/2
  AngleCount_and_EncoderReset/2(Cnt) -> AngleCount/1, Unit Delay1/1
  Bus Selector1/1 -> Compute Distance/1(R), Direction/1(R)  "<R>"
  Bus Selector1/2 -> Compute Distance/2(L), Direction/2(L)  "<L>"
  EC/1 -> Bus Selector1/1
  AngleCount_and_EncoderReset/1(EC) -> Sum/2
  Sum/1 -> EncoderReseted/1
  Compute Distance/1(EncoderMean) -> [Distance], Distance/1, JudgeByDistance/2(Distance), Sum/1, AngleCount_and_EncoderReset/1(In1)
  [AngleCount] -> JudgeByDistance/1(AngleCount)
  JudgeByAngle/1(CountEvent) -> Logical Operator1/1
  JudgeByDistance/1(CountEvent) -> Logical Operator1/2
  Direction/1(Angle) -> Sum2/1
  StartAngle/1 -> Sum2/2
  Logical Operator1/1 -> Logical Operator2/2, Switch/3
  Switch/1 -> AngleCount_and_EncoderReset/Trigger
  Compare To Constant/1 -> Switch/2
  [AngleCount] -> Compare To Constant/1
  Logical Operator2/1 -> Switch/1
  Constant7/1 -> Relational Operator2/1
  Relational Operator2/1 -> Logical Operator2/1
  [Distance] -> Relational Operator2/2

== system et_robocon_princess_pi/Main Controller/normal_operation_modes.line_tracking_mode/line_tracking_mode.Track.lineTracker/Handler ==
  steering : Inport
  fwd : Inport  Port=2
  Constant1 : Constant  Value=-1  OutDataTypeStr=int8
  Mux : Mux  Inputs=2
  Switch1 : Switch  OutDataTypeStr=single  RndMeth=Simplest
  rocket_start : Subsystem
  slow_start : Subsystem
  cmd : Outport
  wires:
  steering/1 -> Mux/2  "str"
  slow_start/1(fwd_slow) -> Switch1/1
  Mux/1 -> cmd/1
  fwd/1 -> rocket_start/1(fwd), slow_start/1(fwd)  "fwd"
  Constant1/1 -> Switch1/2
  rocket_start/1(fwd_slow) -> Switch1/3
  Switch1/1 -> Mux/1

== system et_robocon_princess_pi/Main Controller/normal_operation_modes.line_tracking_mode/line_tracking_mode.Track.lineTracker/SwitchForFreeSteering ==
  note: Edge Change
      | -1: Run right edge
      | 1: Run left edge
  note: Target Value
  FlagSteering : Inport
  PID : Inport  Port=2  PortDimensions=5
  LightSens : Inport  Port=3
  Add : Sum  Inputs=+-  AccumDataTypeStr=single  OutDataTypeStr=single  RndMeth=Simplest
  AdjustForUnit : Gain  Gain=18.25  OutDataTypeStr=single  RndMeth=Simplest
  Constant2 : Constant  OutDataTypeStr=single  SampleTime=-1
  Constant6 : Constant  Value=0.5  OutDataTypeStr=single  SampleTime=-1
  DeleteDummyData : Selector  InputPortWidth=5  IndexOptions=Index vector (dialog)  Indices=1  OutputSizes=1
  Product1 : Product  OutDataTypeStr=single  RndMeth=Simplest
  Switch : Switch  Criteria=u2 > Threshold
  tmpController : Subsystem  TreatAsAtomicUnit=on  mask(tmp PID Controller){Ts_=ts2, SaturationMax=100, SaturationMin=-100}
      mask prompts: Ts_ "Sampling Time (Task Period)"; SaturationMax "Saturation Max Value of PID Ctrl"; SaturationMin "Saturation Min Value of PID"
      mask help:
      | Sampling Time: Task Period
      | P: Proportional Gain
      | I: Integral Gain
      | D: Derivative Gain
      | B: Back Gain for Integrator
      | Saturation Max Value of PID ctrl:
      |    Saturation Max Value of PID ctrl > Saturation Min Value of PID ctrl
      | Saturation Min Value of PID ctrl:
      |    Saturation Min Value of PID ctrl < Saturation Max Value of PID ctrl
      settings: RTWSystemCode=Inline
      mask Display: disp('PID')
  Steering : Outport
  wires:
  PID/1 -> tmpController/2(BD), DeleteDummyData/1
  Switch/1 -> Steering/1
  DeleteDummyData/1 -> Switch/1  "FreeSteering"
  FlagSteering/1 -> Switch/2
  Add/1 -> Product1/1
  LightSens/1 -> Add/1
  Constant6/1 -> Add/2
  Constant2/1 -> Product1/2
  Product1/1 -> tmpController/1(Error)  "Diff_Between_Target_and_Value"
  tmpController/1(Target_deg) -> AdjustForUnit/1
  AdjustForUnit/1 -> Switch/3  "LintTraceSteering"

== system et_robocon_princess_pi/Main Controller/normal_operation_modes.line_tracking_mode/line_tracking_mode.Track.processLight/OFF2ON ==
  In1 : Inport
  Trigger : TriggerPort
  Light Sensor Switch ON : S-Function  FunctionName=sfun_light_sw  Parameters=-1,ip,sw  EnableBusSupport=off  mask(Light Sensor ON/OFF Switch){ip=S3, sw=ON}
      mask prompts: ip "port:"; sw "switch"
      mask help: LEGO Mindstorms NXT Light Sensor switch.
      mask init:
      | [data, map]=imread('LIGHT_SENSOR.gif');
      | pic=ind2rgb(data,map);
      mask TypeOptions ip: S1 | S2 | S3 | S4
      mask TypeOptions sw: ON | OFF
      mask Display:
      | image(pic)
      | color('red')
      | fprintf('%s, %s',ip,sw)
  Out1 : Outport
  wires:
  In1/1 -> Out1/1

== system et_robocon_princess_pi/Main Controller/normal_operation_modes.line_tracking_mode/line_tracking_mode.Track.processLight/ON2OFF ==
  In1 : Inport
  Trigger : TriggerPort  TriggerType=falling
  Light Sensor Switch OFF : S-Function  FunctionName=sfun_light_sw  Parameters=-1,ip,sw  EnableBusSupport=off  mask(Light Sensor ON/OFF Switch){ip=S3, sw=OFF}
      mask prompts: ip "port:"; sw "switch"
      mask help: LEGO Mindstorms NXT Light Sensor switch.
      mask init:
      | [data, map]=imread('LIGHT_SENSOR.gif');
      | pic=ind2rgb(data,map);
      mask TypeOptions ip: S1 | S2 | S3 | S4
      mask TypeOptions sw: ON | OFF
      mask Display:
      | image(pic)
      | color('red')
      | fprintf('%s, %s',ip,sw)
  Out1 : Outport
  wires:
  In1/1 -> Out1/1

== system et_robocon_princess_pi/Main Controller/normal_operation_modes.line_tracking_mode/line_tracking_mode.balanceControl/ForSimulation ==
  cmd_forward : Inport
  cmd_turn : Inport  Port=2
  gyro : Inport  Port=3
  gyro_offset : Inport  Port=4
  theta_m_l : Inport  Port=5
  theta_m_r : Inport  Port=6
  battery : Inport  Port=7
  Cal_PWM : Subsystem
      settings: RTWSystemCode=Nonreusable function
  Cal_Reference : Subsystem  Description=|
      | 1111111111111111111
      | 2222222222222222222
      | 3333333333333333333
      | 4444444444444444444
      settings: RTWSystemCode=Nonreusable function
  Cal_x1 : Subsystem
      settings: RTWSystemCode=Nonreusable function
  DiscreteIntegrator : Subsystem
  FeedbackGain : Gain  Gain=k_f  Multiplication=Matrix(K*u)  OutDataTypeStr=Inherit: Same as input  ParamDataTypeStr=Inherit: Same as input
  IntegralGain : Gain  Gain=k_i  Multiplication=Matrix(K*u)  OutDataTypeStr=Inherit: Same as input  ParamDataTypeStr=Inherit: Same as input
  Sum1 : Sum  Inputs=|+-  OutDataTypeStr=Inherit: Same as first input
  Sum2 : Sum  Inputs=+-|  OutDataTypeStr=Inherit: Same as first input
  sum_err : Sum  Inputs=|++  OutDataTypeStr=Inherit: Same as first input
  pwm_l : Outport
  pwm_r : Outport  Port=2
  wires:
  Cal_Reference/1(pwm_turn) -> Cal_PWM/1(pwm_turn)
  cmd_turn/1 -> Cal_Reference/2(cmd_turn)
  sum_err/1 -> Cal_PWM/2(err)
  FeedbackGain/1 -> sum_err/2  "errx1"
  Cal_Reference/2(theta_ref) -> Sum1/1
  Cal_x1/1(theta) -> Sum1/2
  Sum1/1 -> DiscreteIntegrator/1(in)
  DiscreteIntegrator/1(out) -> IntegralGain/1
  IntegralGain/1 -> sum_err/1  "errtheta"
  Cal_x1/2(x1) -> Sum2/2
  Sum2/1 -> FeedbackGain/1
  Cal_Reference/3(x1_ref) -> Sum2/1
  theta_m_l/1 -> Cal_x1/3(theta_m_l)
  theta_m_r/1 -> Cal_x1/4(theta_m_r)
  cmd_forward/1 -> Cal_Reference/1(cmd_forward)
  Cal_PWM/1(pwm_l) -> pwm_l/1
  gyro/1 -> Cal_x1/1(gyro)
  Cal_PWM/2(pwm_r) -> pwm_r/1
  gyro_offset/1 -> Cal_x1/2(gyro_offset)
  battery/1 -> Cal_PWM/3(battery)

== system et_robocon_princess_pi/Main Controller/normal_operation_modes.line_tracking_mode/line_tracking_mode.balanceControl/Low Pass Filter ==
  u : Inport
  Constant : Constant  Value=0  OutDataTypeStr=boolean
  Low Pass Filter : DiscreteFilter  Numerator=[.01]  Denominator=[1 -0.99]
  Memory : Memory  X0=1  InheritSampleTime=on
  Store Offset : Subsystem  TreatAsAtomicUnit=on
  Sum1 : Sum  Inputs=++|
  Sum2 : Sum  Inputs=-+|
  y : Outport
  wires:
  Store Offset/1(x0) -> Sum1/1, Sum2/1
  u/1 -> Store Offset/1(x), Sum2/2
  Constant/1 -> Memory/1
  Memory/1 -> Store Offset/Enable
  Sum2/1 -> Low Pass Filter/1
  Sum1/1 -> y/1
  Low Pass Filter/1 -> Sum1/2

== system et_robocon_princess_pi/Main Controller/normal_operation_modes.see_saw_princess/see_saw_mode.lineTracker/LPF and deriv ==
  light : Inport
  Discrete Filter : DiscreteFilter  Numerator=[0.05]  Denominator=[1 -0.95]
  Gain : Gain  Gain=1/0.004
  Sum3 : Sum  Inputs=+-
  Unit Delay : UnitDelay  SampleTime=-1
  light_dot : Outport
  wires:
  light/1 -> Discrete Filter/1
  Discrete Filter/1 -> Gain/1
  Sum3/1 -> light_dot/1  "theta_dot_dot"
  Gain/1 -> Sum3/1, Unit Delay/1
  Unit Delay/1 -> Sum3/2

== system et_robocon_princess_pi/State Estimation/Data Type Conversion Unit Conversion Tail Initialization/Low Pass Filter ==
  u : Inport
  Constant : Constant  Value=0  OutDataTypeStr=boolean
  Low Pass Filter : DiscreteFilter  Numerator=[.01]  Denominator=[1 -0.99]
  Memory : Memory  X0=1  InheritSampleTime=on
  Store Offset : Subsystem  TreatAsAtomicUnit=on
  Sum1 : Sum  Inputs=++|
  Sum2 : Sum  Inputs=-+|
  y : Outport
  wires:
  Store Offset/1(x0) -> Sum1/1, Sum2/1
  u/1 -> Store Offset/1(x), Sum2/2
  Constant/1 -> Memory/1
  Memory/1 -> Store Offset/Enable
  Sum2/1 -> Low Pass Filter/1
  Sum1/1 -> y/1
  Low Pass Filter/1 -> Sum1/2

== system et_robocon_princess_pi/State Estimation/Data Type Conversion Unit Conversion Tail Initialization/Process Sonar ==
  sonar_in : Inport
  Constant : Constant  Value=single(255)
  Logical Operator : Logic  Inputs=4  AllPortsSameDT=off  OutDataTypeStr=boolean
  Logical Operator1 : Logic  Operator=NOT  AllPortsSameDT=off  OutDataTypeStr=boolean
  Rate Transition : RateTransition  OutPortSampleTime=0.02
  Rate Transition1 : RateTransition  OutPortSampleTime=0.004
  Relational Operator{,1..3} (4 alike) : RelationalOperator  Operator===  OutDataTypeStr=boolean
  Switch : Switch  Criteria=u2 ~= 0
  Unit Delay{,1..3} (4 alike) : UnitDelay  SampleTime=-1
  sonar : Outport
  wires:
  Switch/1 -> sonar/1  "sonar"
  Constant/1 -> Switch/3
  Rate Transition1/1 -> Switch/2
  Logical Operator1/1 -> Rate Transition1/1
  Logical Operator/1 -> Logical Operator1/1
  Relational Operator2/1 -> Logical Operator/3
  Relational Operator1/1 -> Logical Operator/2
  Relational Operator3/1 -> Logical Operator/4
  Relational Operator/1 -> Logical Operator/1
  Unit Delay3/1 -> Relational Operator3/2
  Unit Delay2/1 -> Unit Delay3/1, Relational Operator2/2, Relational Operator3/1
  Unit Delay1/1 -> Unit Delay2/1, Relational Operator1/2, Relational Operator2/1
  Unit Delay/1 -> Unit Delay1/1, Relational Operator/2, Relational Operator1/1
  Rate Transition/1 -> Unit Delay/1, Relational Operator/1
  sonar_in/1 -> Rate Transition/1, Switch/1

== system et_robocon_princess_pi/State Estimation/Data Type Conversion Unit Conversion Tail Initialization/Vmax ==
  Battery : Inport
  Constant : Constant  Value=0.625  OutDataTypeStr=single
  Gain1 : Gain  Gain=0.001089
  Sum : Sum  Inputs=|+-
  Vmax : Outport
  wires:
  Battery/1 -> Gain1/1
  Gain1/1 -> Sum/1
  Constant/1 -> Sum/2
  Sum/1 -> Vmax/1

== system et_robocon_princess_pi/State Estimation/Data Type Conversion Unit Conversion Tail Initialization/tail processing ==
  sensors : Inport
  init_tail : Inport  Port=2
  Sum : Sum  Inputs=-+|
  tail initialization : Subsystem  TreatAsAtomicUnit=on
  tail : Outport  OutputWhenDisabled=reset  InitialOutput=0
  wires:
  Sum/1 -> tail/1  "theta_T"
  sensors/1 -> Sum/2, tail initialization/1(tail)
  tail initialization/1(tail_0) -> Sum/1
  init_tail/1 -> tail initialization/Trigger

== system et_robocon_princess_pi/State Estimation/Gyro Processing/Compute psi ==
  gyro : Inport
  Trigger : TriggerPort  TriggerType=function-call  StatesWhenEnabling=reset  PortDimensions=1
  Discrete-Time Integrator : DiscreteIntegrator  SampleTime=-1  ICPrevOutput=DiscIntNeverNeededParam  ICPrevScaledInput=DiscIntNeverNeededParam
  Discrete-Time Integrator1 : DiscreteIntegrator  SampleTime=-1  ICPrevOutput=DiscIntNeverNeededParam  ICPrevScaledInput=DiscIntNeverNeededParam
  Sum3 : Sum  Inputs=|+-
  Very Low Pass Filter : Subsystem
  psi : Outport  InitialOutput=0
  Filtered : Outport  Port=2  InitialOutput=0
  wires:
  Discrete-Time Integrator/1 -> Filtered/1
  Discrete-Time Integrator1/1 -> psi/1
  Sum3/1 -> Discrete-Time Integrator/1
  Very Low Pass Filter/1(Out1) -> Sum3/2
  gyro/1 -> Very Low Pass Filter/1(In1), Sum3/1, Discrete-Time Integrator1/1

== system et_robocon_princess_pi/State Estimation/Gyro Processing/Gyro initialization ==
  gyro : Inport
  Enable : EnablePort  StatesWhenEnabling=reset
  Low Pass Filter : DiscreteFilter  Numerator=[.01]  Denominator=[1 -0.99]
  psi_dot_0 : Outport  InitialOutput=0
  wires:
  Low Pass Filter/1 -> psi_dot_0/1
  gyro/1 -> Low Pass Filter/1
